simulink model "FIR_RealizedModelTest"  (R2020b)
settings: Solver=VariableStepAuto  StartTime=0.0  StopTime=10.0  RelTol=1e-3
undefined symbols (not defined in the file): designMultirateFIR
libraries: dspsnks4 x1, dspmlti4 x1, dspvision x1
settings Model: Creator=amira  LastModifiedBy=amira

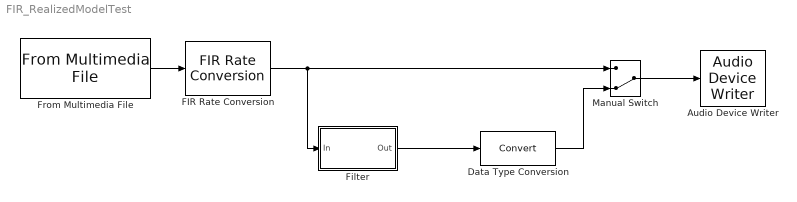
== system FIR_RealizedModelTest ==
  Audio Device Writer : dspsnks4/Audio Device Writer  Driver=DirectSound  Device=Default  InheritSampleRate=on  SampleRate=44100  BitDepth=16-bit integer  BufferSize=4096  NumBuffers=10  DefaultOutputChannelMapping=on  OutputChannelMapping=1:2  OutputNumUnderrunSamples=off  DriverIdx=1  DeviceWarnFlag=''
  Data Type Conversion : DataTypeConversion
  FIR Rate Conversion : dspmlti4/FIR Rate Conversion  FilterSource=Auto  L=160  h=designMultirateFIR(3,2)  M=147  FilterObject=FRC  rateMode=Enforce single-rate processing  roundingMode=Floor  overflowMode=off  firstCoeffDataTypeStr=Inherit: Same word length as input  firstCoeffMin=[]  firstCoeffMax=[]  firstCoeffLastDataTypeStr=Inherit: Same word length as input  outputDataTypeStr=Inherit: Same as accumulator  outputMin=[]  outputMax=[]  outputLastDataTypeStr=Inherit: Same as accumulator
      settings: SourceProductBaseCode=DS
  Filter : Subsystem  Tag=BlockMethodSubSystem
  From Multimedia File : dspvision/From Multimedia File  inputFilename=C:\Classes\semester 7\FPGA\LAB\3\آزمایش سوم-20221129\input.wav  readRange=[1 Inf]  loop=on  numPlays=inf  outputStreams=Audio only  videoDataType=single  audioDataType=double  inheritSampleTime=on  userDefinedSampleTime=1/30  noAudioOutput=off  isIntensityVideo=off  fourcc=RGB  colorVideoFormat=Separate color signals  outputEOF=off  dataOrg=Column-major  audioFrameSize=1470  computeAudioFrameSize=off  outSamplingMode=Sample based
  Manual Switch : ManualSwitch  CurrentSetting=0
  wires:
  From Multimedia File/1 -> FIR Rate Conversion/1
  FIR Rate Conversion/1 -> Filter/1(In), Manual Switch/1
  Manual Switch/1 -> Audio Device Writer/1
  Filter/1(Out) -> Data Type Conversion/1
  Data Type Conversion/1 -> Manual Switch/2

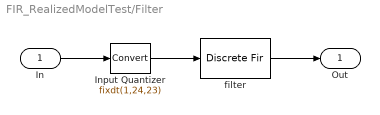
== system FIR_RealizedModelTest/Filter ==
  In : Inport
  Input Quantizer : DataTypeConversion  OutDataTypeStr=fixdt(1,24,23)  RndMeth=Round  SaturateOnIntegerOverflow=on
  filter : DiscreteFir  Coefficients=[-0.00199770033737375332 -0.0050522246581640208 -0.00833204912297771071 -0.0105388507214209063 -0.00928605369156703178 -0.00465626636433711001 0.00212771748052050305 0.00721999616778091439 0.00780919715731914505 0.00275559566900015823 -0.00484572504694240781 -0.0102132088672959379 -0.00881394373220143607 -0.000690352173205861092 0.00960397765611908927 0.0146313292123977159 0.00973684132692750892 -0.00361887609436985962 -0.0170513010495714941 -0.0205544961577479764 -0.0090655570931518388 0.0122143910511979866 0.0296448351798478012 0.0287131289736472783 0.00469944790841886426 -0.0315005469808854605 -0.056127791025032292 -0.0446362691219116606 0.0137655672079026545 0.106967350932166139 0.202872902404592215 0.263502567263083076 0.263502567263083076 0.202872902404592215 0.106967350932166139 0.0137655672079026545 -0.0446362691219116606 -0.056127791025032292 -0.0315005469808854605 0.00469944790841886426 0.0287131289736472783 0.0296448351798478012 0.0122143910511979866 -0.0090655570931518388 -0.0205544961577479764 -0.0170513010495714941 -0.00361887609436985962 0.00973684132692750892 0.0146313292123977159 0.00960397765611908927 -0.000690352173205861092 -0.00881394373220143607 -0.0102132088672959379 -0.00484572504694240781 0.00275559566900015823 0.00780919715731914505 0.00721999616778091439 0.00212771748052050305 -0.00465626636433711001 -0.00928605369156703178 -0.0105388507214209063 -0.00833204912297771071 -0.0050522246581640208 -0.00199770033737375332]  InputProcessing=Columns as channels (frame based)  CoefDataTypeStr=fixdt(true,16,16)  ProductDataTypeStr=fixdt(true,31,31)  AccumDataTypeStr=fixdt(true,34,31)  OutDataTypeStr=fixdt(true,32,30)  RndMeth=Convergent
  Out : Outport
  wires:
  In/1 -> Input Quantizer/1
  Input Quantizer/1 -> filter/1
  filter/1 -> Out/1
